simulink model "ADCS_Simulator"  (R2025b)
settings: Solver=ode4  StartTime=0.0  StopTime=tspan  FixedStep=baseRate  RelTol=1e-3
values from neighbouring files (symbols this model uses):
  A_list = [10*30; 10*30; 10*10; 10*30; 10*30; 10*10] * 1e-04    [adcsInitializer.m]
  A_w = eye(3)    [adcsInitializer.m]
  CD = 2.3    [adcsInitializer.m]
  COP = [xAxis/2   0          0 ... (first row only)    [adcsInitializer.m]
  dt = 0.5    [adcsInitializer.m]
  dYear = decyear(YYYY,MM,DD)    [adcsInitializer.m]
  eta = 0.3    [adcsInitializer.m]
  J_body = [ I_xx  I_xy  I_xz ... (first row only)    [adcsInitializer.m]
  mag_moment = [0.005; 0.005; 0.005]    [adcsInitializer.m]
  mu = 398600.4418    [adcsInitializer.m]    (also in montecarlo.m = mean(W,2))
  n_list = [1 0 0; 0 1 0; 0 0 1; -1 0 0; 0 -1 0; 0 0 -1]    [adcsInitializer.m]
  p = 0.00000451    (= 4.51e-06)    [adcsInitializer.m]
  R = blkdiag(sigma_S^2*eye(3), sigma_B^2*eye(3))    [adcsInitializer.m]
  rE = 6378.14    [adcsInitializer.m]
  sigma_b = deg2rad(0.04)/3600    [adcsInitializer.m]
  sigma_B = 0.001    [adcsInitializer.m]
  sigma_g = deg2rad(0.1)/sqrt(3600)    [adcsInitializer.m]
  sigma_S = deg2rad(0.01)    [adcsInitializer.m]
  T = 1    [adcsInitializer.m]
  wE = [0 0 15.04*(pi/180)*(1/3600)]    [adcsInitializer.m]
  wW_1 = 0    [adcsInitializer.m]
  wW_2 = 0    [adcsInitializer.m]
  wW_3 = 0    [adcsInitializer.m]
undefined symbols (not defined in the file or in its folder): ar, controlMode, ext_torque, J_wheels, K_d, K_p, K_w, n, period, pointingMode, q1_ini, q2_ini, q3_ini, q4_ini, r_I_ini, sigmaGPS, turns, useFilter, v_I_ini, wB_1, wB_2, wB_3
libraries: simulink_extras x12
(part 1 of 2)
settings Model: Creator=nimis  LastModifiedBy=nimis

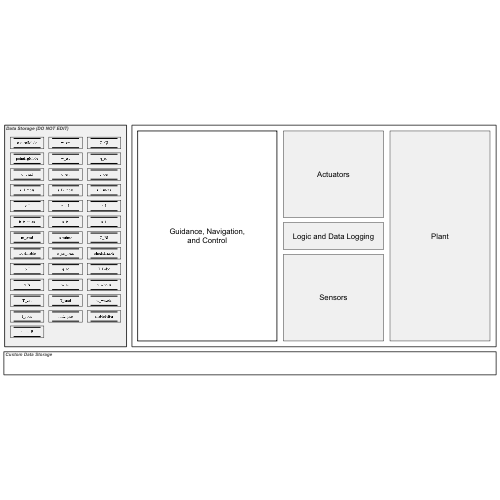
[thumbnail: Simulink's stored preview of the top-level diagram]
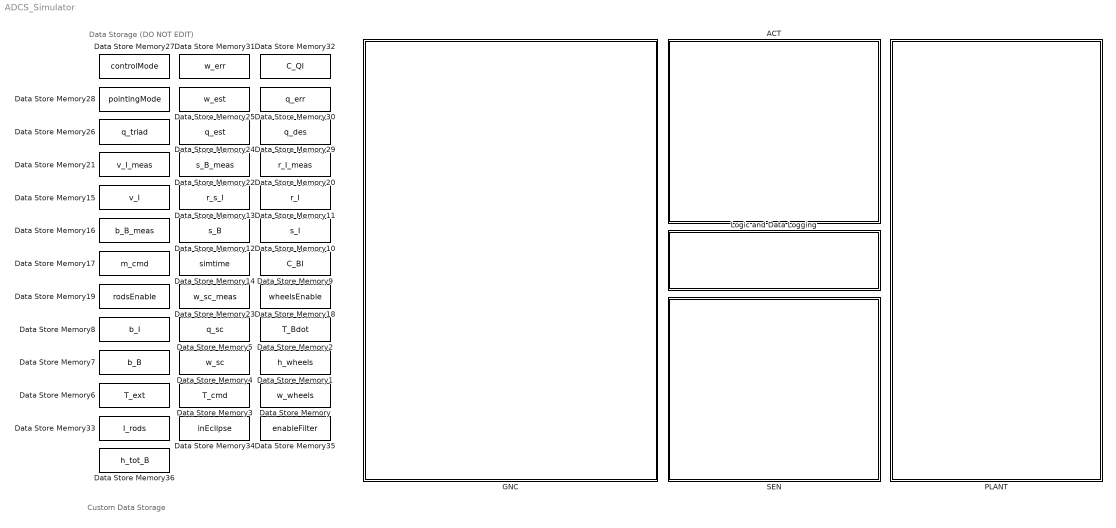
== system ADCS_Simulator ==
  note: Custom Data Storage
  note: Data Storage (DO NOT EDIT)
  ACT : Subsystem
      mask Display: disp('Actuators');
  Data Store Memory : DataStoreMemory  DataStoreName=w_wheels  WriteAfterWriteMsg=warning  InitialValue=[0;0;0]  ShowAdditionalParam=off
  Data Store Memory1 : DataStoreMemory  DataStoreName=h_wheels  WriteAfterWriteMsg=warning  InitialValue=[0;0;0]  ShowAdditionalParam=off
  Data Store Memory10 : DataStoreMemory  DataStoreName=s_I  WriteAfterWriteMsg=warning  InitialValue=[0;0;0]  ShowAdditionalParam=off
  Data Store Memory11 : DataStoreMemory  DataStoreName=r_I  WriteAfterWriteMsg=warning  InitialValue=r_I_ini  ShowAdditionalParam=off
  Data Store Memory12 : DataStoreMemory  DataStoreName=s_B  WriteAfterWriteMsg=warning  InitialValue=[0;0;0]  ShowAdditionalParam=off
  Data Store Memory13 : DataStoreMemory  DataStoreName=r_s_I  WriteAfterWriteMsg=warning  InitialValue=[0;0;0]  ShowAdditionalParam=off
  Data Store Memory14 : DataStoreMemory  DataStoreName=simtime  WriteAfterWriteMsg=warning  ShowAdditionalParam=off
  Data Store Memory15 : DataStoreMemory  DataStoreName=v_I  WriteAfterWriteMsg=warning  InitialValue=v_I_ini  ShowAdditionalParam=off
  Data Store Memory16 : DataStoreMemory  DataStoreName=b_B_meas  WriteAfterWriteMsg=warning  InitialValue=[0;0;0]  ShowAdditionalParam=off
  Data Store Memory17 : DataStoreMemory  DataStoreName=m_cmd  WriteAfterWriteMsg=warning  InitialValue=[0;0;0]  ShowAdditionalParam=off
  Data Store Memory18 : DataStoreMemory  DataStoreName=wheelsEnable  WriteAfterWriteMsg=warning  ShowAdditionalParam=off
  Data Store Memory19 : DataStoreMemory  DataStoreName=rodsEnable  WriteAfterWriteMsg=warning  InitialValue=1  ShowAdditionalParam=off
  Data Store Memory2 : DataStoreMemory  DataStoreName=T_Bdot  WriteAfterWriteMsg=warning  InitialValue=[0;0;0]  ShowAdditionalParam=off
  Data Store Memory20 : DataStoreMemory  DataStoreName=r_I_meas  WriteAfterWriteMsg=warning  InitialValue=r_I_ini  ShowAdditionalParam=off
  Data Store Memory21 : DataStoreMemory  DataStoreName=v_I_meas  WriteAfterWriteMsg=warning  InitialValue=v_I_ini  ShowAdditionalParam=off
  Data Store Memory22 : DataStoreMemory  DataStoreName=s_B_meas  WriteAfterWriteMsg=warning  InitialValue=[0;0;0]  ShowAdditionalParam=off
  Data Store Memory23 : DataStoreMemory  DataStoreName=w_sc_meas  WriteAfterWriteMsg=warning  InitialValue=[wB_1; wB_2; wB_3]*(pi/180)  ShowAdditionalParam=off
  Data Store Memory24 : DataStoreMemory  DataStoreName=q_est  WriteAfterWriteMsg=warning  InitialValue=[q1_ini; q2_ini; q3_ini; q4_ini]  ShowAdditionalParam=off
  Data Store Memory25 : DataStoreMemory  DataStoreName=w_est  WriteAfterWriteMsg=warning  InitialValue=[wB_1; wB_2; wB_3]*(pi/180)  ShowAdditionalParam=off
  Data Store Memory26 : DataStoreMemory  DataStoreName=q_triad  WriteAfterWriteMsg=warning  InitialValue=[q1_ini; q2_ini; q3_ini; q4_ini]  ShowAdditionalParam=off
  Data Store Memory27 : DataStoreMemory  DataStoreName=controlMode  WriteAfterWriteMsg=warning  InitialValue=controlMode  ShowAdditionalParam=off
  Data Store Memory28 : DataStoreMemory  DataStoreName=pointingMode  WriteAfterWriteMsg=warning  InitialValue=pointingMode  ShowAdditionalParam=off
  Data Store Memory29 : DataStoreMemory  DataStoreName=q_des  WriteAfterWriteMsg=warning  InitialValue=[0;0;0;0]  ShowAdditionalParam=off
  Data Store Memory3 : DataStoreMemory  DataStoreName=T_cmd  WriteAfterWriteMsg=warning  InitialValue=[0;0;0]  ShowAdditionalParam=off
  Data Store Memory30 : DataStoreMemory  DataStoreName=q_err  WriteAfterWriteMsg=warning  InitialValue=[0;0;0;1]  ShowAdditionalParam=off
  Data Store Memory31 : DataStoreMemory  DataStoreName=w_err  WriteAfterWriteMsg=warning  InitialValue=[0;0;0]  ShowAdditionalParam=off
  Data Store Memory32 : DataStoreMemory  DataStoreName=C_QI  WriteAfterWriteMsg=warning  InitialValue=eye(3)  ShowAdditionalParam=off
  Data Store Memory33 : DataStoreMemory  DataStoreName=I_rods  WriteAfterWriteMsg=warning  InitialValue=[0;0;0]  ShowAdditionalParam=off
  Data Store Memory34 : DataStoreMemory  DataStoreName=inEclipse  WriteAfterWriteMsg=warning  ShowAdditionalParam=off
  Data Store Memory35 : DataStoreMemory  DataStoreName=enableFilter  WriteAfterWriteMsg=warning  InitialValue=double(useFilter)  ShowAdditionalParam=off
      settings: LockScale=on
  Data Store Memory36 : DataStoreMemory  DataStoreName=h_tot_B  WriteAfterWriteMsg=warning  InitialValue=[0;0;0]  ShowAdditionalParam=off
  Data Store Memory4 : DataStoreMemory  DataStoreName=w_sc  WriteAfterWriteMsg=warning  InitialValue=[wB_1; wB_2; wB_3]*(pi/180)  ShowAdditionalParam=off
  Data Store Memory5 : DataStoreMemory  DataStoreName=q_sc  WriteAfterWriteMsg=warning  InitialValue=[q1_ini; q2_ini; q3_ini; q4_ini]  ShowAdditionalParam=off
  Data Store Memory6 : DataStoreMemory  DataStoreName=T_ext  WriteAfterWriteMsg=warning  InitialValue=[0;0;0]  ShowAdditionalParam=off
  Data Store Memory7 : DataStoreMemory  DataStoreName=b_B  WriteAfterWriteMsg=warning  InitialValue=[0;0;0]  ShowAdditionalParam=off
  Data Store Memory8 : DataStoreMemory  DataStoreName=b_I  WriteAfterWriteMsg=warning  InitialValue=[0;0;0]  ShowAdditionalParam=off
  Data Store Memory9 : DataStoreMemory  DataStoreName=C_BI  WriteAfterWriteMsg=warning  InitialValue=eye(3)  ShowAdditionalParam=off
  GNC : Subsystem  TreatAsAtomicUnit=on  SystemSampleTime=dt
      mask Display: disp('Guidance, Navigation,\nand Control');
  Logic and Data Logging : Subsystem
      mask Display: disp('Logic and Data Logging');
  PLANT : Subsystem
      mask Display: disp('Plant');
  SEN : Subsystem
      mask Display: disp('Sensors');

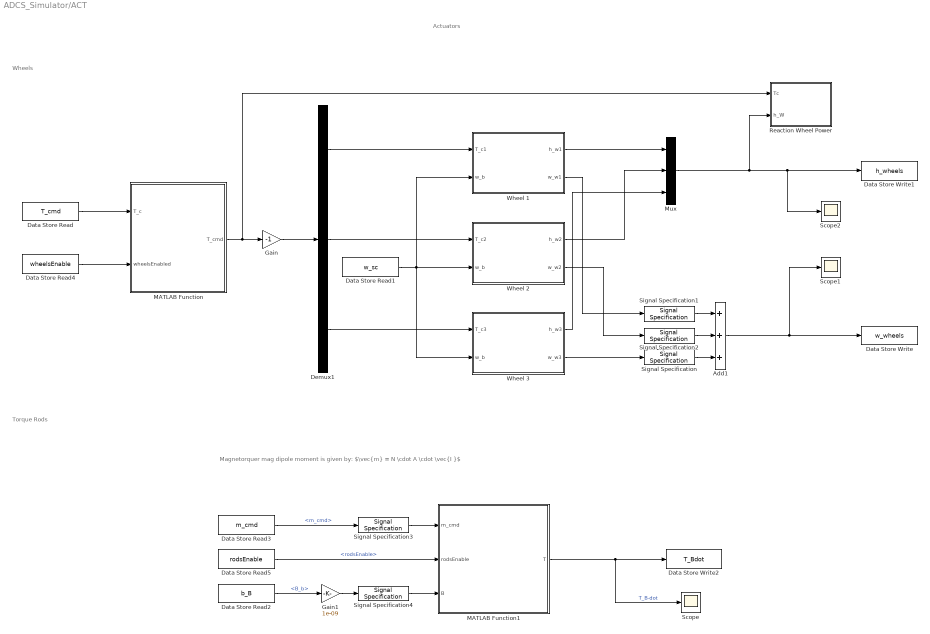
== system ADCS_Simulator/ACT ==
  note: Torque Rods
  note: Wheels
  note: Actuators
  note: Magnetorquer mag dipole moment is given by:
      | $\vec{m} = N \cdot A \cdot \vec{I }$
  Add1 : Sum  Inputs=+++
  Data Store Read : DataStoreRead  DataStoreName=T_cmd  IndexOptions=Index vector (dialog)  Indices=1  OutputSizes=1
  Data Store Read1 : DataStoreRead  DataStoreName=w_sc  IndexOptions=Index vector (dialog)  Indices=1  OutputSizes=1
  Data Store Read2 : DataStoreRead  DataStoreName=b_B  IndexOptions=Index vector (dialog)  Indices=1  OutputSizes=1
  Data Store Read3 : DataStoreRead  DataStoreName=m_cmd  IndexOptions=Index vector (dialog)  Indices=1  OutputSizes=1
  Data Store Read4 : DataStoreRead  DataStoreName=wheelsEnable  IndexOptions=Index vector (dialog)  Indices=1  OutputSizes=1
  Data Store Read5 : DataStoreRead  DataStoreName=rodsEnable  IndexOptions=Index vector (dialog)  Indices=1  OutputSizes=1
  Data Store Write : DataStoreWrite  DataStoreName=w_wheels  IndexOptions=Index vector (dialog)  Indices=1  OutputSizes=1
  Data Store Write1 : DataStoreWrite  DataStoreName=h_wheels  IndexOptions=Index vector (dialog)  Indices=1  OutputSizes=1
  Data Store Write2 : DataStoreWrite  DataStoreName=T_Bdot  IndexOptions=Index vector (dialog)  Indices=1  OutputSizes=1
  Demux1 : Demux  Outputs=3
  Gain : Gain  Gain=-1
  Gain1 : Gain  Gain=1e-09
  MATLAB Function : MATLAB Function  TreatAsAtomicUnit=on
  MATLAB Function1 : MATLAB Function  TreatAsAtomicUnit=on
  Mux : Mux  Inputs=3
  Reaction Wheel Power : Subsystem
  Scope : Scope
      settings: ActiveDisplayYMinimum=-1  ActiveDisplayYMaximum=1  DataLoggingVariableName=ScopeData2
  Scope1 : Scope
      settings: ActiveDisplayYMinimum=-0.2676  ActiveDisplayYMaximum=2.40696
  Scope2 : Scope
      settings: ActiveDisplayYMinimum=-0.00052  ActiveDisplayYMaximum=0.00026
  Signal Specification{,1..4} (5 alike) : SignalSpecification  Dimensions=[3,1]
  Wheel 1 : Subsystem
  Wheel 2 : Subsystem
  Wheel 3 : Subsystem
  wires:
  Data Store Read1/1 -> Wheel 1/2(w_b), Wheel 2/2(w_b), Wheel 3/2(w_b)
  Gain/1 -> Demux1/1
  Wheel 1/2(w_w1) -> Signal Specification1/1
  Demux1/2 -> Wheel 2/1(T_c2)
  Data Store Read4/1 -> MATLAB Function/2(wheelsEnabled)
  Wheel 3/1(h_w3) -> Mux/3
  Wheel 1/1(h_w1) -> Mux/1
  Demux1/1 -> Wheel 1/1(T_c1)
  Data Store Read/1 -> MATLAB Function/1(T_c)
  Signal Specification1/1 -> Add1/1
  Signal Specification2/1 -> Add1/2
  Add1/1 -> Data Store Write/1, Scope1/1
  Wheel 2/1(h_w2) -> Mux/2
  Mux/1 -> Scope2/1, Data Store Write1/1, Reaction Wheel Power/2(h_W)
  Wheel 3/2(w_w3) -> Signal Specification/1
  Demux1/3 -> Wheel 3/1(T_c3)
  Wheel 2/2(w_w2) -> Signal Specification2/1
  MATLAB Function/1(T_cmd) -> Gain/1, Reaction Wheel Power/1(Tc)
  Signal Specification/1 -> Add1/3
  Data Store Read3/1 -> Signal Specification3/1  "<m_cmd>"
  Data Store Read2/1 -> Gain1/1  "<B_b>"
  Signal Specification4/1 -> MATLAB Function1/3(B)
  Signal Specification3/1 -> MATLAB Function1/1(m_cmd)
  Data Store Read5/1 -> MATLAB Function1/2(rodsEnable)  "<rodsEnable>"
  MATLAB Function1/1(T) -> Data Store Write2/1, Scope/1  "T_B-dot"
  Gain1/1 -> Signal Specification4/1

== system ADCS_Simulator/GNC ==
  note: Guidance, Navigation, and Control
  Control : Subsystem
  Data Store Write10 : DataStoreWrite  DataStoreName=m_cmd  IndexOptions=Index vector (dialog)  Indices=1  OutputSizes=1
  Data Store Write9 : DataStoreWrite  DataStoreName=T_cmd  IndexOptions=Index vector (dialog)  Indices=1  OutputSizes=1
  Guidance : Subsystem
  Navigation : Subsystem
  wires:
  Navigation/1(q_est) -> Guidance/1(q_body)
  Navigation/2(w_est) -> Guidance/2(w_body)
  Control/1(T_cmd) -> Data Store Write9/1
  Control/2(m_cmd) -> Data Store Write10/1

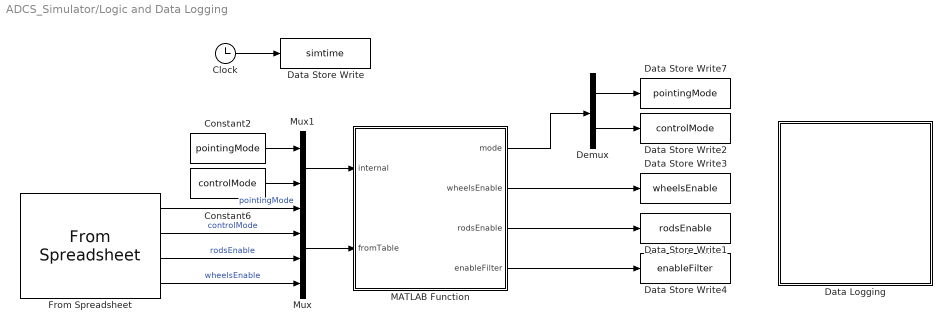
== system ADCS_Simulator/Logic and Data Logging ==
  Clock : Clock
  Constant2 : Constant  Value=pointingMode
  Constant6 : Constant  Value=controlMode
  Data Logging : Subsystem
  Data Store Write : DataStoreWrite  DataStoreName=simtime  IndexOptions=Index vector (dialog)  Indices=1  OutputSizes=1
  Data Store Write1 : DataStoreWrite  DataStoreName=rodsEnable  IndexOptions=Index vector (dialog)  Indices=1  OutputSizes=1
  Data Store Write2 : DataStoreWrite  DataStoreName=controlMode  IndexOptions=Index vector (dialog)  Indices=1  OutputSizes=1
  Data Store Write3 : DataStoreWrite  DataStoreName=wheelsEnable  IndexOptions=Index vector (dialog)  Indices=1  OutputSizes=1
  Data Store Write4 : DataStoreWrite  DataStoreName=enableFilter  IndexOptions=Index vector (dialog)  Indices=1  OutputSizes=1
  Data Store Write7 : DataStoreWrite  DataStoreName=pointingMode  IndexOptions=Index vector (dialog)  Indices=1  OutputSizes=1
  Demux : Demux  Outputs=2
  From Spreadsheet : FromSpreadsheet  FileName=controlCommand.xlsx  SheetName=commands  Range=B1:F1000  InterpolationWithinTimeRange=Zero order hold  ExtrapolationAfterLastDataPoint=Hold last value
  MATLAB Function : MATLAB Function  TreatAsAtomicUnit=on
  Mux : Mux
  Mux1 : Mux  Inputs=2
  wires:
  Clock/1 -> Data Store Write/1
  MATLAB Function/3(rodsEnable) -> Data Store Write1/1
  Mux/1 -> MATLAB Function/2(fromTable)
  From Spreadsheet/1 -> Mux/1  "pointingMode"
  Mux1/1 -> MATLAB Function/1(internal)
  MATLAB Function/2(wheelsEnable) -> Data Store Write3/1
  From Spreadsheet/3 -> Mux/3  "rodsEnable"
  From Spreadsheet/2 -> Mux/2  "controlMode"
  Constant2/1 -> Mux1/1
  Constant6/1 -> Mux1/2
  Demux/1 -> Data Store Write7/1
  Demux/2 -> Data Store Write2/1
  MATLAB Function/4(enableFilter) -> Data Store Write4/1
  From Spreadsheet/4 -> Mux/4  "wheelsEnable"
  MATLAB Function/1(mode) -> Demux/1

== system ADCS_Simulator/PLANT ==
  note: PLANT
  Data Store Read3 : DataStoreRead  DataStoreName=h_wheels  IndexOptions=Index vector (dialog)  Indices=1  OutputSizes=1
  Data Store Read4 : DataStoreRead  DataStoreName=T_Bdot  IndexOptions=Index vector (dialog)  Indices=1  OutputSizes=1
  Data Store Read5 : DataStoreRead  DataStoreName=T_ext  IndexOptions=Index vector (dialog)  Indices=1  OutputSizes=1
  Data Store Write : DataStoreWrite  DataStoreName=T_ext  IndexOptions=Index vector (dialog)  Indices=1  OutputSizes=1
  Data Store Write3 : DataStoreWrite  DataStoreName=w_sc  IndexOptions=Index vector (dialog)  Indices=1  OutputSizes=1
  Data Store Write4 : DataStoreWrite  DataStoreName=q_sc  IndexOptions=Index vector (dialog)  Indices=1  OutputSizes=1
  ENV : Subsystem  Priority=4  VariantControl=ext_torque == true
  Orbit Propator : Subsystem  Priority=3
  Spacecraft Dynamics : Subsystem  Priority=1
  Spacecraft Kinematics : Subsystem  Priority=2
  wires:
  ENV/1(T_ext) -> Data Store Write/1
  Data Store Read5/1 -> Spacecraft Dynamics/2(T_ext)
  Spacecraft Kinematics/1(q) -> Data Store Write4/1
  Data Store Read3/1 -> Spacecraft Dynamics/1(h_w)
  Spacecraft Dynamics/1(w_b) -> Data Store Write3/1, Spacecraft Kinematics/1(w)
  Data Store Read4/1 -> Spacecraft Dynamics/3(T_Bdot)

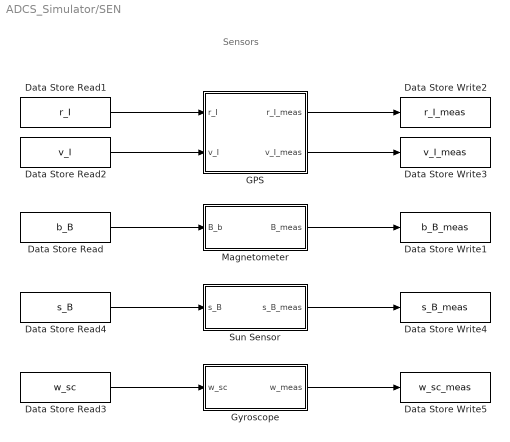
== system ADCS_Simulator/SEN ==
  note: Sensors
  Data Store Read : DataStoreRead  DataStoreName=b_B  IndexOptions=Index vector (dialog)  Indices=1  OutputSizes=1
  Data Store Read1 : DataStoreRead  DataStoreName=r_I  IndexOptions=Index vector (dialog)  Indices=1  OutputSizes=1
  Data Store Read2 : DataStoreRead  DataStoreName=v_I  IndexOptions=Index vector (dialog)  Indices=1  OutputSizes=1
  Data Store Read3 : DataStoreRead  DataStoreName=w_sc  IndexOptions=Index vector (dialog)  Indices=1  OutputSizes=1
  Data Store Read4 : DataStoreRead  DataStoreName=s_B  IndexOptions=Index vector (dialog)  Indices=1  OutputSizes=1
  Data Store Write1 : DataStoreWrite  DataStoreName=b_B_meas  IndexOptions=Index vector (dialog)  Indices=1  OutputSizes=1
  Data Store Write2 : DataStoreWrite  DataStoreName=r_I_meas  IndexOptions=Index vector (dialog)  Indices=1  OutputSizes=1
  Data Store Write3 : DataStoreWrite  DataStoreName=v_I_meas  IndexOptions=Index vector (dialog)  Indices=1  OutputSizes=1
  Data Store Write4 : DataStoreWrite  DataStoreName=s_B_meas  IndexOptions=Index vector (dialog)  Indices=1  OutputSizes=1
  Data Store Write5 : DataStoreWrite  DataStoreName=w_sc_meas  IndexOptions=Index vector (dialog)  Indices=1  OutputSizes=1
  GPS : Subsystem
  Gyroscope : Subsystem
  Magnetometer : Subsystem
  Sun Sensor : Subsystem
  wires:
  GPS/1(r_I_meas) -> Data Store Write2/1
  GPS/2(v_I_meas) -> Data Store Write3/1
  Magnetometer/1(B_meas) -> Data Store Write1/1
  Sun Sensor/1(s_B_meas) -> Data Store Write4/1
  Gyroscope/1(w_meas) -> Data Store Write5/1
  Data Store Read1/1 -> GPS/1(r_I)
  Data Store Read2/1 -> GPS/2(v_I)
  Data Store Read/1 -> Magnetometer/1(B_b)
  Data Store Read4/1 -> Sun Sensor/1(s_B)
  Data Store Read3/1 -> Gyroscope/1(w_sc)

== system ADCS_Simulator/ACT/Reaction Wheel Power ==
  Tc : Inport
  h_W : Inport  Port=2
  MATLAB Function3 : MATLAB Function  TreatAsAtomicUnit=on
  Scope2 : Scope
      settings: ActiveDisplayYMinimum=-170.39311  ActiveDisplayYMaximum=1533.53798  DataLoggingVariableName=ScopeData2
  Scope4 : Scope
      settings: ActiveDisplayYMinimum=-0.0048  ActiveDisplayYMaximum=0.04316
  To Workspace : ToWorkspace  VariableName=Prw  SampleTime=-1
  Unit Delay : UnitDelay  InitialCondition=zeros(3,1)  SampleTime=-1  HasFrameUpgradeWarning=on
  wires:
  MATLAB Function3/1(Prw) -> To Workspace/1, Scope4/1
  Tc/1 -> MATLAB Function3/1(Tc)
  MATLAB Function3/2(Ptotal) -> Unit Delay/1, Scope2/1
  h_W/1 -> MATLAB Function3/2(h_W)
  Unit Delay/1 -> MATLAB Function3/3(P_pre)

== system ADCS_Simulator/ACT/Wheel 1 ==
  T_c1 : Inport
  w_b : Inport  Port=2
  Constant1 : Constant  Value=A_w
  Constant2 : Constant  Value=J_wheels
  Integrator1 : Integrator  InitialCondition=wW_1*J_wheels
  MATLAB Function1 : MATLAB Function  TreatAsAtomicUnit=on
  Reshape : Reshape  OutputDimensionality=Column vector (2-D)
  Transfer Fcn : TransferFcn  Commented=on  Numerator=[2.11e04]  Denominator=[J_wheels 1 0]
  Transfer Fcn (with initial states) : simulink_extras/Additional Linear/Transfer Fcn (with initial states)  Commented=on  N=[1]  D="[T  1]"  X0=wW_1*J_wheels
  h_w1 : Outport
  w_w1 : Outport  Port=2
  wires:
  Constant2/1 -> MATLAB Function1/1(J_w)
  T_c1/1 -> Integrator1/1
  w_b/1 -> Reshape/1
  Constant1/1 -> MATLAB Function1/4(A_w)
  MATLAB Function1/1(h_wi) -> h_w1/1
  MATLAB Function1/2(w_wi) -> w_w1/1
  Integrator1/1 -> MATLAB Function1/2(h_w)
  Reshape/1 -> MATLAB Function1/3(wB)

== system ADCS_Simulator/ACT/Wheel 2 ==
  T_c2 : Inport
  w_b : Inport  Port=2
  Constant2 : Constant  Value=A_w
  Constant3 : Constant  Value=J_wheels
  Integrator1 : Integrator  InitialCondition=wW_2*J_wheels
  MATLAB Function1 : MATLAB Function  TreatAsAtomicUnit=on
  Reshape : Reshape  OutputDimensionality=Column vector (2-D)
  Transfer Fcn : TransferFcn  Commented=on  Numerator=[2.11e04]  Denominator=[J_wheels 1 0]
  Transfer Fcn (with initial states) : simulink_extras/Additional Linear/Transfer Fcn (with initial states)  Commented=on  N=[1]  D="[T  1]"  X0=wW_2*J_wheels
  h_w2 : Outport
  w_w2 : Outport  Port=2
  wires:
  Constant2/1 -> MATLAB Function1/4(A_w)
  T_c2/1 -> Integrator1/1
  Constant3/1 -> MATLAB Function1/1(J_w)
  MATLAB Function1/2(w_wi) -> w_w2/1
  Integrator1/1 -> MATLAB Function1/2(h_w)
  MATLAB Function1/1(h_wi) -> h_w2/1
  w_b/1 -> Reshape/1
  Reshape/1 -> MATLAB Function1/3(wB)

== system ADCS_Simulator/ACT/Wheel 3 ==
  T_c3 : Inport
  w_b : Inport  Port=2
  Constant2 : Constant  Value=A_w
  Constant3 : Constant  Value=J_wheels
  Integrator1 : Integrator  InitialCondition=wW_3*J_wheels
  MATLAB Function1 : MATLAB Function  TreatAsAtomicUnit=on
  Reshape : Reshape  OutputDimensionality=Column vector (2-D)
  Transfer Fcn : TransferFcn  Commented=on  Numerator=[2.11e04]  Denominator=[J_wheels 1 0]
  Transfer Fcn (with initial states) : simulink_extras/Additional Linear/Transfer Fcn (with initial states)  Commented=on  N=[1]  D="[T  1]"  X0=wW_3*J_wheels
  h_w3 : Outport
  w_w3 : Outport  Port=2
  wires:
  Constant2/1 -> MATLAB Function1/4(A_w)
  T_c3/1 -> Integrator1/1
  Constant3/1 -> MATLAB Function1/1(J_w)
  MATLAB Function1/2(w_wi) -> w_w3/1
  Integrator1/1 -> MATLAB Function1/2(h_w)
  MATLAB Function1/1(h_wi) -> h_w3/1
  w_b/1 -> Reshape/1
  Reshape/1 -> MATLAB Function1/3(wB)

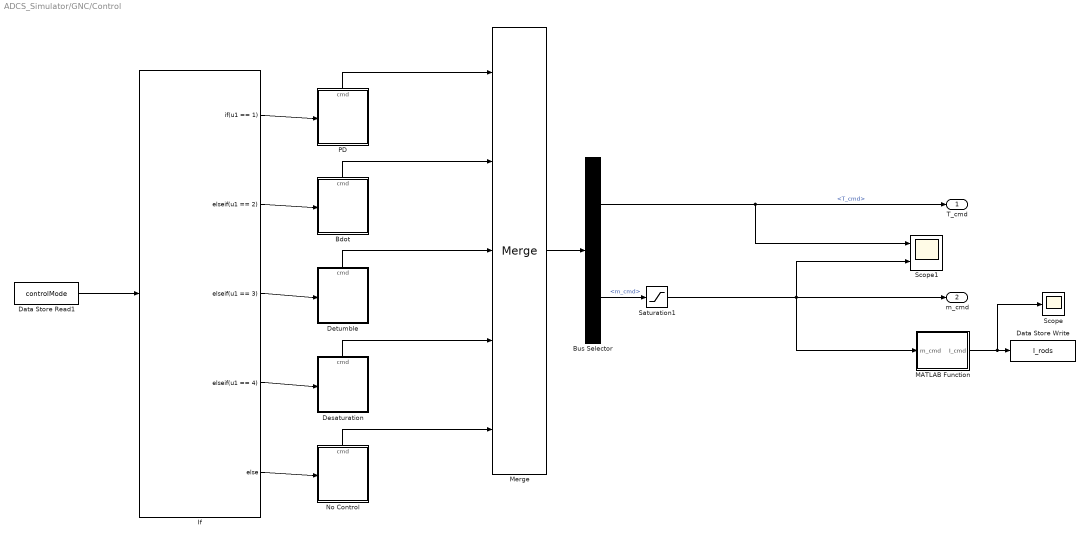
== system ADCS_Simulator/GNC/Control ==
  Bdot : Subsystem  TreatAsAtomicUnit=on
  Bus Selector : BusSelector  OutputSignals=T_cmd,m_cmd
  Data Store Read1 : DataStoreRead  DataStoreName=controlMode  IndexOptions=Index vector (dialog)  Indices=1  OutputSizes=1
  Data Store Write : DataStoreWrite  DataStoreName=I_rods  IndexOptions=Index vector (dialog)  Indices=1  OutputSizes=1
  Desaturation : Subsystem  TreatAsAtomicUnit=on
  Detumble : Subsystem  TreatAsAtomicUnit=on
  If : If  IfExpression=u1 == 1  ElseIfExpressions=u1 == 2, u1 == 3, u1 == 4
  MATLAB Function : MATLAB Function  TreatAsAtomicUnit=on
  Merge : Merge  Inputs=5
  No Control : Subsystem  TreatAsAtomicUnit=on
  "PD " : Subsystem  TreatAsAtomicUnit=on
  Saturation1 : Saturate  UpperLimit=0.2  LowerLimit=-0.2
  Scope : Scope
      settings: ActiveDisplayYMinimum=-1  ActiveDisplayYMaximum=1  DataLoggingVariableName=ScopeData2
  Scope1 : Scope  NumInputPorts=2
      settings: ActiveDisplayYMinimum=-7.0811470476357021E-5  ActiveDisplayYMaximum=7.7475119642045185E-5  DataLoggingVariableName=ScopeData4
  T_cmd : Outport
  m_cmd : Outport  Port=2
  wires:
  If/1 -> "PD "/Action
  If/2 -> Bdot/Action
  If/3 -> Detumble/Action
  If/4 -> Desaturation/Action
  If/5 -> No Control/Action
  Data Store Read1/1 -> If/1
  "PD "/1(cmd) -> Merge/1
  Bdot/1(cmd) -> Merge/2
  Detumble/1(cmd) -> Merge/3
  Desaturation/1(cmd) -> Merge/4
  No Control/1(cmd) -> Merge/5
  Merge/1 -> Bus Selector/1
  Saturation1/1 -> MATLAB Function/1(m_cmd), Scope1/2, m_cmd/1
  Bus Selector/2 -> Saturation1/1  "<m_cmd>"
  Bus Selector/1 -> T_cmd/1, Scope1/1  "<T_cmd>"
  MATLAB Function/1(I_cmd) -> Scope/1, Data Store Write/1

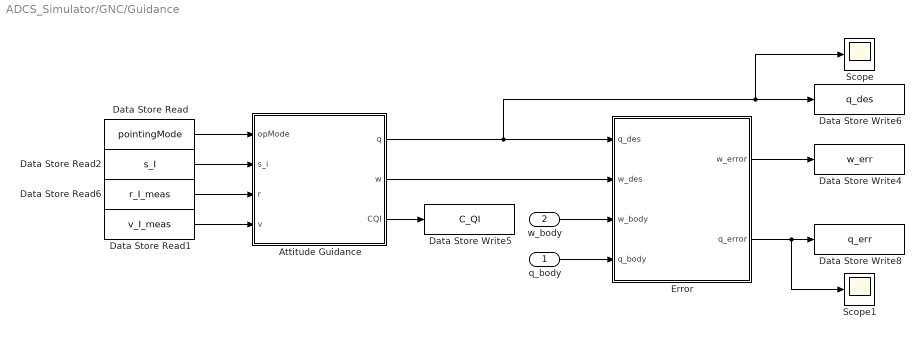
== system ADCS_Simulator/GNC/Guidance ==
  q_body : Inport
  w_body : Inport  Port=2
  Attitude Guidance : MATLAB Function  TreatAsAtomicUnit=on
  Data Store Read : DataStoreRead  DataStoreName=pointingMode  IndexOptions=Index vector (dialog)  Indices=1  OutputSizes=1
  Data Store Read1 : DataStoreRead  DataStoreName=v_I_meas  IndexOptions=Index vector (dialog)  Indices=1  OutputSizes=1
  Data Store Read2 : DataStoreRead  DataStoreName=s_I  IndexOptions=Index vector (dialog)  Indices=1  OutputSizes=1
  Data Store Read6 : DataStoreRead  DataStoreName=r_I_meas  IndexOptions=Index vector (dialog)  Indices=1  OutputSizes=1
  Data Store Write4 : DataStoreWrite  DataStoreName=w_err  IndexOptions=Index vector (dialog)  Indices=1  OutputSizes=1
  Data Store Write5 : DataStoreWrite  DataStoreName=C_QI  IndexOptions=Index vector (dialog)  Indices=1  OutputSizes=1
  Data Store Write6 : DataStoreWrite  DataStoreName=q_des  IndexOptions=Index vector (dialog)  Indices=1  OutputSizes=1
  Data Store Write8 : DataStoreWrite  DataStoreName=q_err  IndexOptions=Index vector (dialog)  Indices=1  OutputSizes=1
  Error : Subsystem
  Scope : Scope
      settings: ActiveDisplayYMinimum=-1.056652169354914  ActiveDisplayYMaximum=0.82334453801197993
  Scope1 : Scope
      settings: ActiveDisplayYMinimum=-1  ActiveDisplayYMaximum=1  DataLoggingVariableName=ScopeData2
  wires:
  Error/2(q_error) -> Scope1/1, Data Store Write8/1
  Data Store Read/1 -> Attitude Guidance/1(opMode)
  Data Store Read6/1 -> Attitude Guidance/3(r)
  Data Store Read2/1 -> Attitude Guidance/2(s_i)
  Error/1(w_error) -> Data Store Write4/1
  Attitude Guidance/3(CQI) -> Data Store Write5/1
  q_body/1 -> Error/4(q_body)
  Data Store Read1/1 -> Attitude Guidance/4(v)
  w_body/1 -> Error/3(w_body)
  Attitude Guidance/2(w) -> Error/2(w_des)
  Attitude Guidance/1(q) -> Error/1(q_des), Scope/1, Data Store Write6/1

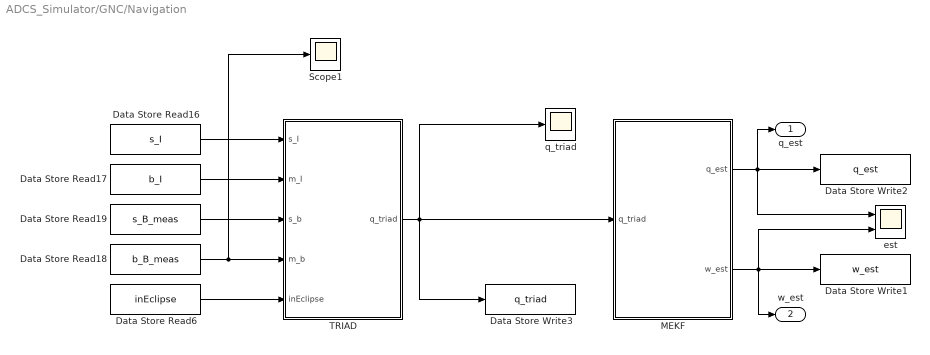
== system ADCS_Simulator/GNC/Navigation ==
  Data Store Read16 : DataStoreRead  DataStoreName=s_I  IndexOptions=Index vector (dialog)  Indices=1  OutputSizes=1
  Data Store Read17 : DataStoreRead  DataStoreName=b_I  IndexOptions=Index vector (dialog)  Indices=1  OutputSizes=1
  Data Store Read18 : DataStoreRead  DataStoreName=b_B_meas  IndexOptions=Index vector (dialog)  Indices=1  OutputSizes=1
  Data Store Read19 : DataStoreRead  DataStoreName=s_B_meas  IndexOptions=Index vector (dialog)  Indices=1  OutputSizes=1
  Data Store Read6 : DataStoreRead  DataStoreName=inEclipse  IndexOptions=Index vector (dialog)  Indices=1  OutputSizes=1
  Data Store Write1 : DataStoreWrite  DataStoreName=w_est  IndexOptions=Index vector (dialog)  Indices=1  OutputSizes=1
  Data Store Write2 : DataStoreWrite  DataStoreName=q_est  IndexOptions=Index vector (dialog)  Indices=1  OutputSizes=1
  Data Store Write3 : DataStoreWrite  DataStoreName=q_triad  IndexOptions=Index vector (dialog)  Indices=1  OutputSizes=1
  MEKF : Subsystem
  Scope1 : Scope
      settings: ActiveDisplayYMinimum=-14383.00265  ActiveDisplayYMaximum=50097.51975
  TRIAD : MATLAB Function  TreatAsAtomicUnit=on
  est : Scope  NumInputPorts=2
      settings: ActiveDisplayYMinimum=-1.1965212617720182  ActiveDisplayYMaximum=1.242899979906531
  q_triad : Scope
      settings: ActiveDisplayYMinimum=-1.09993445466622  ActiveDisplayYMaximum=1.2333260505184689  DataLoggingVariableName=ScopeData3
  q_est : Outport
  w_est : Outport  Port=2
  wires:
  Data Store Read19/1 -> TRIAD/3(s_b)
  MEKF/2(w_est) -> w_est/1, Data Store Write1/1, est/2
  MEKF/1(q_est) -> q_est/1, Data Store Write2/1, est/1
  Data Store Read18/1 -> Scope1/1, TRIAD/4(m_b)
  Data Store Read17/1 -> TRIAD/2(m_I)
  TRIAD/1(q_triad) -> Data Store Write3/1, q_triad/1, MEKF/1(q_triad)
  Data Store Read16/1 -> TRIAD/1(s_I)
  Data Store Read6/1 -> TRIAD/5(inEclipse)

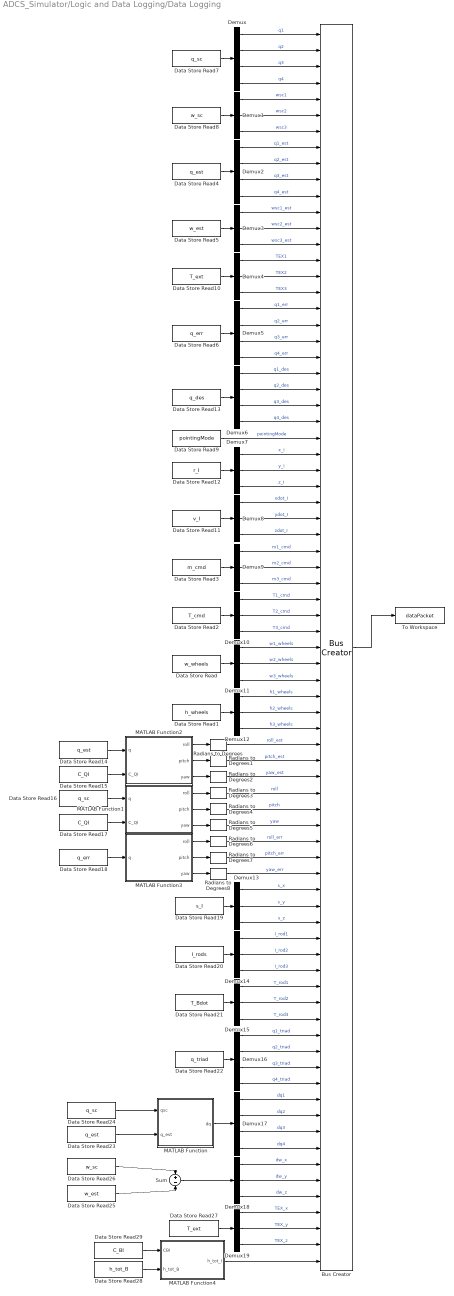
== system ADCS_Simulator/Logic and Data Logging/Data Logging ==
  Bus Creator : BusCreator  Inputs=77
  Data Store Read : DataStoreRead  DataStoreName=w_wheels  IndexOptions=Index vector (dialog)  Indices=1  OutputSizes=1
  Data Store Read1 : DataStoreRead  DataStoreName=h_wheels  IndexOptions=Index vector (dialog)  Indices=1  OutputSizes=1
  Data Store Read10 : DataStoreRead  DataStoreName=T_ext  IndexOptions=Index vector (dialog)  Indices=1  OutputSizes=1
  Data Store Read11 : DataStoreRead  DataStoreName=v_I  IndexOptions=Index vector (dialog)  Indices=1  OutputSizes=1
  Data Store Read12 : DataStoreRead  DataStoreName=r_I  IndexOptions=Index vector (dialog)  Indices=1  OutputSizes=1
  Data Store Read13 : DataStoreRead  DataStoreName=q_des  IndexOptions=Index vector (dialog)  Indices=1  OutputSizes=1
  Data Store Read14 : DataStoreRead  DataStoreName=q_est  IndexOptions=Index vector (dialog)  Indices=1  OutputSizes=1
  Data Store Read15 : DataStoreRead  DataStoreName=C_QI  IndexOptions=Index vector (dialog)  Indices=1  OutputSizes=1
  Data Store Read16 : DataStoreRead  DataStoreName=q_sc  IndexOptions=Index vector (dialog)  Indices=1  OutputSizes=1
  Data Store Read17 : DataStoreRead  DataStoreName=C_QI  IndexOptions=Index vector (dialog)  Indices=1  OutputSizes=1
  Data Store Read18 : DataStoreRead  DataStoreName=q_err  IndexOptions=Index vector (dialog)  Indices=1  OutputSizes=1
  Data Store Read19 : DataStoreRead  DataStoreName=s_I  IndexOptions=Index vector (dialog)  Indices=1  OutputSizes=1
  Data Store Read2 : DataStoreRead  DataStoreName=T_cmd  IndexOptions=Index vector (dialog)  Indices=1  OutputSizes=1
  Data Store Read20 : DataStoreRead  DataStoreName=I_rods  IndexOptions=Index vector (dialog)  Indices=1  OutputSizes=1
  Data Store Read21 : DataStoreRead  DataStoreName=T_Bdot  IndexOptions=Index vector (dialog)  Indices=1  OutputSizes=1
  Data Store Read22 : DataStoreRead  DataStoreName=q_triad  IndexOptions=Index vector (dialog)  Indices=1  OutputSizes=1
  Data Store Read23 : DataStoreRead  DataStoreName=q_est  IndexOptions=Index vector (dialog)  Indices=1  OutputSizes=1
  Data Store Read24 : DataStoreRead  DataStoreName=q_sc  IndexOptions=Index vector (dialog)  Indices=1  OutputSizes=1
  Data Store Read25 : DataStoreRead  DataStoreName=w_est  IndexOptions=Index vector (dialog)  Indices=1  OutputSizes=1
  Data Store Read26 : DataStoreRead  DataStoreName=w_sc  IndexOptions=Index vector (dialog)  Indices=1  OutputSizes=1
  Data Store Read27 : DataStoreRead  DataStoreName=T_ext  IndexOptions=Index vector (dialog)  Indices=1  OutputSizes=1
  Data Store Read28 : DataStoreRead  DataStoreName=h_tot_B  IndexOptions=Index vector (dialog)  Indices=1  OutputSizes=1
  Data Store Read29 : DataStoreRead  DataStoreName=C_BI  IndexOptions=Index vector (dialog)  Indices=1  OutputSizes=1
  Data Store Read3 : DataStoreRead  DataStoreName=m_cmd  IndexOptions=Index vector (dialog)  Indices=1  OutputSizes=1
  Data Store Read4 : DataStoreRead  DataStoreName=q_est  IndexOptions=Index vector (dialog)  Indices=1  OutputSizes=1
  Data Store Read5 : DataStoreRead  DataStoreName=w_est  IndexOptions=Index vector (dialog)  Indices=1  OutputSizes=1
  Data Store Read6 : DataStoreRead  DataStoreName=q_err  IndexOptions=Index vector (dialog)  Indices=1  OutputSizes=1
  Data Store Read7 : DataStoreRead  DataStoreName=q_sc  IndexOptions=Index vector (dialog)  Indices=1  OutputSizes=1
  Data Store Read8 : DataStoreRead  DataStoreName=w_sc  IndexOptions=Index vector (dialog)  Indices=1  OutputSizes=1
  Data Store Read9 : DataStoreRead  DataStoreName=pointingMode  IndexOptions=Index vector (dialog)  Indices=1  OutputSizes=1
  Demux{,2,5..6,16..17} (6 alike) : Demux
  Demux{1,3..4,7..15,18..19} (14 alike) : Demux  Outputs=3
  MATLAB Function : MATLAB Function  TreatAsAtomicUnit=on
  MATLAB Function1 : MATLAB Function  TreatAsAtomicUnit=on
  MATLAB Function2 : MATLAB Function  TreatAsAtomicUnit=on
  MATLAB Function3 : MATLAB Function  TreatAsAtomicUnit=on
  MATLAB Function4 : MATLAB Function  TreatAsAtomicUnit=on
  Radians to Degrees{,1..8} (9 alike) : simulink_extras/Transformations/Radians to Degrees
  Sum : Sum  Inputs=+-
  To Workspace : ToWorkspace  VariableName=dataPacket  SaveFormat=Timeseries  SampleTime=-1
  wires:
  Data Store Read7/1 -> Demux/1
  Demux/1 -> Bus Creator/1  "q1"
  Demux/2 -> Bus Creator/2  "q2"
  Demux/3 -> Bus Creator/3  "q3"
  Demux/4 -> Bus Creator/4  "q4"
  Data Store Read8/1 -> Demux1/1
  Demux1/1 -> Bus Creator/5  "wsc1"
  Demux1/2 -> Bus Creator/6  "wsc2"
  Demux1/3 -> Bus Creator/7  "wsc3"
  Demux2/1 -> Bus Creator/8  "q1_est"
  Demux2/2 -> Bus Creator/9  "q2_est"
  Demux2/3 -> Bus Creator/10  "q3_est"
  Demux2/4 -> Bus Creator/11  "q4_est"
  Data Store Read4/1 -> Demux2/1
  Demux3/1 -> Bus Creator/12  "wsc1_est"
  Demux3/2 -> Bus Creator/13  "wsc2_est"
  Demux3/3 -> Bus Creator/14  "wsc3_est"
  Data Store Read5/1 -> Demux3/1
  Demux4/1 -> Bus Creator/15  "TEX1"
  Demux4/2 -> Bus Creator/16  "TEX2"
  Demux4/3 -> Bus Creator/17  "TEX3"
  Data Store Read10/1 -> Demux4/1
  Demux5/1 -> Bus Creator/18  "q1_err"
  Demux5/2 -> Bus Creator/19  "q2_err"
  Demux5/3 -> Bus Creator/20  "q3_err"
  Demux5/4 -> Bus Creator/21  "q4_err"
  Data Store Read6/1 -> Demux5/1
  Demux6/1 -> Bus Creator/22  "q1_des"
  Demux6/2 -> Bus Creator/23  "q2_des"
  Demux6/3 -> Bus Creator/24  "q3_des"
  Demux6/4 -> Bus Creator/25  "q4_des"
  Data Store Read13/1 -> Demux6/1
  Data Store Read9/1 -> Bus Creator/26  "pointingMode"
  Demux7/1 -> Bus Creator/27  "x_I"
  Demux7/2 -> Bus Creator/28  "y_I"
  Demux7/3 -> Bus Creator/29  "z_I"
  Data Store Read12/1 -> Demux7/1
  Demux8/1 -> Bus Creator/30  "xdot_I"
  Demux8/2 -> Bus Creator/31  "ydot_I"
  Demux8/3 -> Bus Creator/32  "zdot_I"
  Data Store Read11/1 -> Demux8/1
  Demux9/1 -> Bus Creator/33  "m1_cmd"
  Demux9/2 -> Bus Creator/34  "m2_cmd"
  Demux9/3 -> Bus Creator/35  "m3_cmd"
  Data Store Read3/1 -> Demux9/1
  Demux10/1 -> Bus Creator/36  "T1_cmd"
  Demux10/2 -> Bus Creator/37  "T2_cmd"
  Demux10/3 -> Bus Creator/38  "T3_cmd"
  Data Store Read2/1 -> Demux10/1
  Demux11/1 -> Bus Creator/39  "w1_wheels"
  Demux11/2 -> Bus Creator/40  "w2_wheels"
  Demux11/3 -> Bus Creator/41  "w3_wheels"
  Data Store Read/1 -> Demux11/1
  Demux12/1 -> Bus Creator/42  "h1_wheels"
  Demux12/2 -> Bus Creator/43  "h2_wheels"
  Demux12/3 -> Bus Creator/44  "h3_wheels"
  Data Store Read1/1 -> Demux12/1
  Bus Creator/1 -> To Workspace/1
  MATLAB Function2/1(roll) -> Radians to Degrees/1
  MATLAB Function2/3(yaw) -> Radians to Degrees2/1
  MATLAB Function2/2(pitch) -> Radians to Degrees1/1
  Data Store Read14/1 -> MATLAB Function2/1(q)
  Data Store Read15/1 -> MATLAB Function2/2(C_QI)
  Radians to Degrees/1 -> Bus Creator/45  "roll_est"
  Radians to Degrees1/1 -> Bus Creator/46  "pitch_est"
  Radians to Degrees2/1 -> Bus Creator/47  "yaw_est"
  Radians to Degrees5/1 -> Bus Creator/50  "yaw"
  Radians to Degrees4/1 -> Bus Creator/49  "pitch"
  Radians to Degrees3/1 -> Bus Creator/48  "roll"
  Data Store Read17/1 -> MATLAB Function1/2(C_QI)
  Data Store Read16/1 -> MATLAB Function1/1(q)
  MATLAB Function1/2(pitch) -> Radians to Degrees4/1
  MATLAB Function1/3(yaw) -> Radians to Degrees5/1
  MATLAB Function1/1(roll) -> Radians to Degrees3/1
  MATLAB Function3/1(roll) -> Radians to Degrees6/1
  MATLAB Function3/2(pitch) -> Radians to Degrees7/1
  MATLAB Function3/3(yaw) -> Radians to Degrees8/1
  Data Store Read18/1 -> MATLAB Function3/1(q)
  Radians to Degrees6/1 -> Bus Creator/51  "roll_err"
  Radians to Degrees7/1 -> Bus Creator/52  "pitch_err"
  Radians to Degrees8/1 -> Bus Creator/53  "yaw_err"
  Data Store Read19/1 -> Demux13/1
  Demux13/1 -> Bus Creator/54  "s_x"
  Demux13/2 -> Bus Creator/55  "s_y"
  Demux13/3 -> Bus Creator/56  "s_z"
  Data Store Read20/1 -> Demux14/1
  Demux14/1 -> Bus Creator/57  "I_rod1"
  Demux14/2 -> Bus Creator/58  "I_rod2"
  Demux14/3 -> Bus Creator/59  "I_rod3"
  Demux15/1 -> Bus Creator/60  "T_rod1"
  Demux15/2 -> Bus Creator/61  "T_rod2"
  Demux15/3 -> Bus Creator/62  "T_rod3"
  Data Store Read21/1 -> Demux15/1
  Demux16/3 -> Bus Creator/65  "q3_triad"
  Demux16/1 -> Bus Creator/63  "q1_triad"
  Demux16/2 -> Bus Creator/64  "q2_triad"
  Data Store Read22/1 -> Demux16/1
  Demux16/4 -> Bus Creator/66  "q4_triad"
  Demux17/1 -> Bus Creator/67  "dq1"
  Demux17/2 -> Bus Creator/68  "dq2"
  Demux17/3 -> Bus Creator/69  "dq3"
  Demux17/4 -> Bus Creator/70  "dq4"
  Demux18/1 -> Bus Creator/71  "dw_x"
  Demux18/2 -> Bus Creator/72  "dw_y"
  Demux18/3 -> Bus Creator/73  "dw_z"
  MATLAB Function/1(dq) -> Demux17/1
  Data Store Read24/1 -> MATLAB Function/1(qsc)
  Data Store Read23/1 -> MATLAB Function/2(q_est)
  Data Store Read26/1 -> Sum/1
  Data Store Read25/1 -> Sum/2
  Sum/1 -> Demux18/1
  Demux19/1 -> Bus Creator/74  "TEX_x"
  Demux19/2 -> Bus Creator/75  "TEX_y"
  Demux19/3 -> Bus Creator/76  "TEX_z"
  Data Store Read27/1 -> Demux19/1
  Data Store Read29/1 -> MATLAB Function4/1(CBI)
  Data Store Read28/1 -> MATLAB Function4/2(h_tot_B)
  MATLAB Function4/1(h_tot_I) -> Bus Creator/77

== system ADCS_Simulator/PLANT/ENV ==
  Constant : Constant  Value=ext_torque
  If : If  IfExpression=u1 == 1
  Merge : Merge
  Perturbations Disabled : Subsystem  TreatAsAtomicUnit=on
  Perturbations Enabled : Subsystem  TreatAsAtomicUnit=on
  T_ext : Outport
  wires:
  Constant/1 -> If/1
  If/1 -> Perturbations Enabled/Action
  If/2 -> Perturbations Disabled/Action
  Perturbations Enabled/1(Out1) -> Merge/1
  Perturbations Disabled/1(Out1) -> Merge/2
  Merge/1 -> T_ext/1

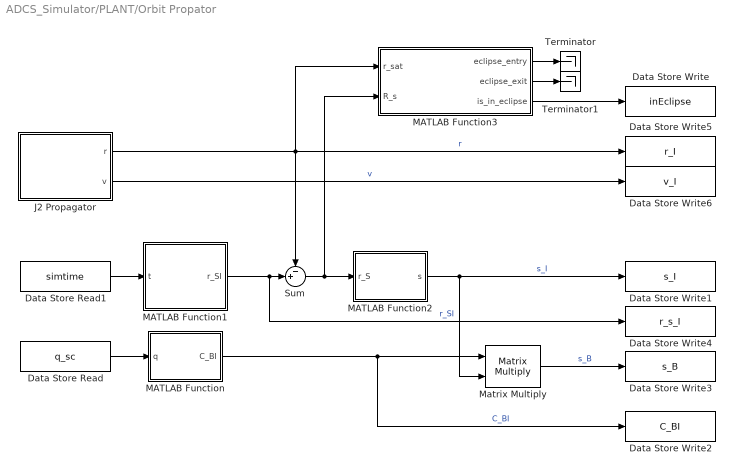
== system ADCS_Simulator/PLANT/Orbit Propator ==
  Data Store Read : DataStoreRead  DataStoreName=q_sc  IndexOptions=Index vector (dialog)  Indices=1  OutputSizes=1
  Data Store Read1 : DataStoreRead  DataStoreName=simtime  IndexOptions=Index vector (dialog)  Indices=1  OutputSizes=1
  Data Store Write : DataStoreWrite  DataStoreName=inEclipse  IndexOptions=Index vector (dialog)  Indices=1  OutputSizes=1
  Data Store Write1 : DataStoreWrite  DataStoreName=s_I  IndexOptions=Index vector (dialog)  Indices=1  OutputSizes=1
  Data Store Write2 : DataStoreWrite  DataStoreName=C_BI  IndexOptions=Index vector (dialog)  Indices=1  OutputSizes=1
  Data Store Write3 : DataStoreWrite  DataStoreName=s_B  IndexOptions=Index vector (dialog)  Indices=1  OutputSizes=1
  Data Store Write4 : DataStoreWrite  DataStoreName=r_s_I  IndexOptions=Index vector (dialog)  Indices=1  OutputSizes=1
  Data Store Write5 : DataStoreWrite  DataStoreName=r_I  IndexOptions=Index vector (dialog)  Indices=1  OutputSizes=1
  Data Store Write6 : DataStoreWrite  DataStoreName=v_I  IndexOptions=Index vector (dialog)  Indices=1  OutputSizes=1
  J2 Propagator : Subsystem
  MATLAB Function : MATLAB Function  TreatAsAtomicUnit=on
  MATLAB Function1 : MATLAB Function  TreatAsAtomicUnit=on
  MATLAB Function2 : MATLAB Function  TreatAsAtomicUnit=on
  MATLAB Function3 : MATLAB Function  TreatAsAtomicUnit=on
  Matrix Multiply : Product  Multiplication=Matrix(*)
  Sum : Sum  Inputs=-+|
  Terminator : Terminator
  Terminator1 : Terminator
  wires:
  MATLAB Function/1(C_BI) -> Data Store Write2/1, Matrix Multiply/1  "C_BI"
  MATLAB Function2/1(s) -> Data Store Write1/1, Matrix Multiply/2  "s_I"
  J2 Propagator/1(r) -> MATLAB Function3/1(r_sat), Sum/1, Data Store Write5/1  "r"
  Data Store Read/1 -> MATLAB Function/1(q)
  Matrix Multiply/1 -> Data Store Write3/1  "s_B"
  J2 Propagator/2(v) -> Data Store Write6/1  "v"
  Data Store Read1/1 -> MATLAB Function1/1(t)
  MATLAB Function1/1(r_SI) -> Data Store Write4/1, Sum/2  "r_SI"
  MATLAB Function3/2(eclipse_exit) -> Terminator1/1
  Sum/1 -> MATLAB Function3/2(R_s), MATLAB Function2/1(r_S)
  MATLAB Function3/1(eclipse_entry) -> Terminator/1
  MATLAB Function3/3(is_in_eclipse) -> Data Store Write/1

== system ADCS_Simulator/PLANT/Spacecraft Dynamics ==
  h_w : Inport
  T_ext : Inport  Port=2
  T_Bdot : Inport  Port=3
  Data Store Write : DataStoreWrite  DataStoreName=h_tot_B  IndexOptions=Index vector (dialog)  Indices=1  OutputSizes=1
  Integrator2 : Integrator  InitialCondition=J_body * [wB_1; wB_2; wB_3]*(pi/180)
  MATLAB Function1 : MATLAB Function  TreatAsAtomicUnit=on
  Reshape : Reshape  OutputDimensionality=Column vector (2-D)  OutputDimensions=[3,1]
  Scope : Scope
      settings: ActiveDisplayYMinimum=-4.3527039546372842E-7  ActiveDisplayYMaximum=4.1195292762308163E-7
  Sum2 : Sum
  w_b : Outport
  wires:
  h_w/1 -> Reshape/1
  T_ext/1 -> Scope/1, Sum2/1
  T_Bdot/1 -> Sum2/2
  Sum2/1 -> MATLAB Function1/2(T_b)
  Reshape/1 -> MATLAB Function1/3(h_w)
  MATLAB Function1/1(h_tot_dot) -> Integrator2/1
  Integrator2/1 -> Data Store Write/1, MATLAB Function1/1(h_tot)
  MATLAB Function1/2(w_b) -> w_b/1

== system ADCS_Simulator/PLANT/Spacecraft Kinematics ==
  note: $\dot \mathbf \epsilon = \frac{1}{2} \left( \eta \ \mathbf I_{3\times3} + \mathbf\epsilon ^{\times} \right) \\ \dot \eta = - \frac{1}{2} \left(\mathbf \epsilon ^{\mathrm{T}} \ \mathbf\omega \right)$
  w : Inport
  Integrator2 : Integrator  InitialCondition=[q1_ini; q2_ini; q3_ini; q4_ini]
  MATLAB Function1 : MATLAB Function  TreatAsAtomicUnit=on
  Quaternion Normalize1 : MATLAB Function  TreatAsAtomicUnit=on
  q : Outport
  wires:
  w/1 -> MATLAB Function1/2(w)
  MATLAB Function1/1(q_dot) -> Integrator2/1
  Integrator2/1 -> Quaternion Normalize1/1(q), MATLAB Function1/1(q)  "q"
  Quaternion Normalize1/1(q_norm) -> q/1

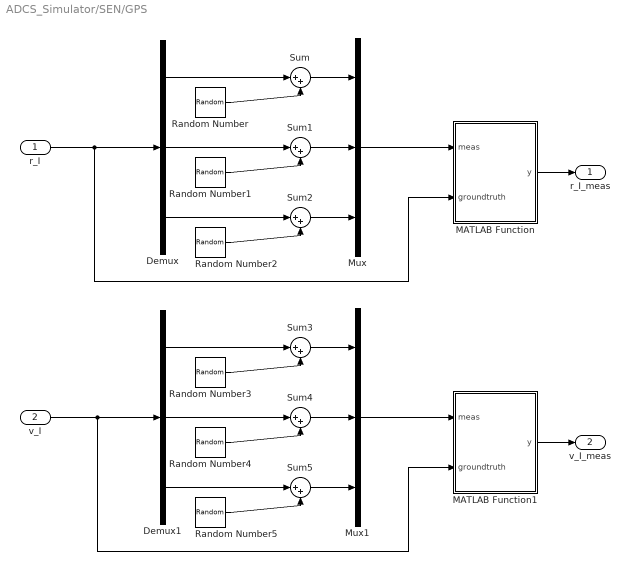
== system ADCS_Simulator/SEN/GPS ==
  r_I : Inport
  v_I : Inport  Port=2
  Demux : Demux  Outputs=3
  Demux1 : Demux  Outputs=3
  MATLAB Function : MATLAB Function  TreatAsAtomicUnit=on
  MATLAB Function1 : MATLAB Function  TreatAsAtomicUnit=on
  Mux : Mux  Inputs=3
  Mux1 : Mux  Inputs=3
  Random Number{,1..5} (6 alike) : RandomNumber  Variance=sigmaGPS^2  Seed=123  SampleTime=1
  Sum{,1..5} (6 alike) : Sum  Inputs=|++
  r_I_meas : Outport
  v_I_meas : Outport  Port=2
  wires:
  Sum1/1 -> Mux/2
  Random Number1/1 -> Sum1/2
  Mux/1 -> MATLAB Function/1(meas)
  Demux/2 -> Sum1/1
  Demux/1 -> Sum/1
  Demux/3 -> Sum2/1
  Sum/1 -> Mux/1
  Sum2/1 -> Mux/3
  Random Number2/1 -> Sum2/2
  r_I/1 -> MATLAB Function/2(groundtruth), Demux/1
  Random Number/1 -> Sum/2
  Mux1/1 -> MATLAB Function1/1(meas)
  v_I/1 -> MATLAB Function1/2(groundtruth), Demux1/1
  Random Number3/1 -> Sum3/2
  Sum4/1 -> Mux1/2
  Sum5/1 -> Mux1/3
  Random Number5/1 -> Sum5/2
  Demux1/1 -> Sum3/1
  Sum3/1 -> Mux1/1
  Random Number4/1 -> Sum4/2
  Demux1/2 -> Sum4/1
  Demux1/3 -> Sum5/1
  MATLAB Function/1(y) -> r_I_meas/1
  MATLAB Function1/1(y) -> v_I_meas/1

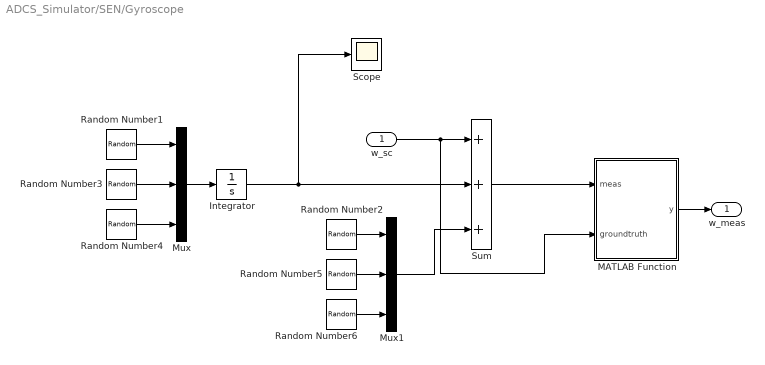
== system ADCS_Simulator/SEN/Gyroscope ==
  w_sc : Inport
  Integrator : Integrator  InitialCondition=1e-09*ones(3,1)
  MATLAB Function : MATLAB Function  TreatAsAtomicUnit=on
  Mux : Mux  Inputs=3
  Mux1 : Mux  Inputs=3
  Random Number1 : RandomNumber  Variance=sigma_b^2  SampleTime=1
  Random Number2 : RandomNumber  Variance=sigma_g^2  SampleTime=1
  Random Number3 : RandomNumber  Variance=sigma_b^2  SampleTime=1
  Random Number4 : RandomNumber  Variance=sigma_b^2  SampleTime=1
  Random Number5 : RandomNumber  Variance=sigma_g^2  SampleTime=1
  Random Number6 : RandomNumber  Variance=sigma_g^2  SampleTime=1
  Scope : Scope
      settings: ActiveDisplayYMinimum=-1  ActiveDisplayYMaximum=1  DataLoggingVariableName=ScopeData2
  Sum : Sum  Inputs=+++
  w_meas : Outport
  wires:
  w_sc/1 -> MATLAB Function/2(groundtruth), Sum/1
  Mux/1 -> Integrator/1
  Random Number1/1 -> Mux/1
  Integrator/1 -> Scope/1, Sum/2
  Mux1/1 -> Sum/3
  Sum/1 -> MATLAB Function/1(meas)
  MATLAB Function/1(y) -> w_meas/1
  Random Number3/1 -> Mux/2
  Random Number4/1 -> Mux/3
  Random Number2/1 -> Mux1/1
  Random Number5/1 -> Mux1/2
  Random Number6/1 -> Mux1/3

== system ADCS_Simulator/SEN/Magnetometer ==
  B_b : Inport
  Demux : Demux  Outputs=3
  MATLAB Function : MATLAB Function  TreatAsAtomicUnit=on
  Mux : Mux  Inputs=3
  Random Number : RandomNumber  Variance=sigma_B^2  Seed=123  SampleTime=1
  Random Number1 : RandomNumber  Variance=sigma_B^2  Seed=123  SampleTime=1
  Random Number2 : RandomNumber  Variance=sigma_B^2  Seed=123  SampleTime=1
  Sum : Sum  Inputs=|++
  Sum1 : Sum  Inputs=|++
  Sum2 : Sum  Inputs=|++
  B_meas : Outport
  wires:
  Mux/1 -> MATLAB Function/1(meas)
  Sum2/1 -> Mux/3
  Random Number/1 -> Sum/2
  Random Number1/1 -> Sum1/2
  Demux/3 -> Sum2/1
  Demux/2 -> Sum1/1
  Sum1/1 -> Mux/2
  Demux/1 -> Sum/1
  Sum/1 -> Mux/1
  Random Number2/1 -> Sum2/2
  MATLAB Function/1(y) -> B_meas/1
  B_b/1 -> MATLAB Function/2(groundtruth), Demux/1

== system ADCS_Simulator/SEN/Sun Sensor ==
  note: This assumes that the sun sensor reference frame coincides
      | with the sc body reference frame
  s_B : Inport
  Data Store Read6 : DataStoreRead  DataStoreName=inEclipse  IndexOptions=Index vector (dialog)  Indices=1  OutputSizes=1
  Demux : Demux  Outputs=3
  MATLAB Function : MATLAB Function  TreatAsAtomicUnit=on
  Mux : Mux  Inputs=3
  Random Number : RandomNumber  Variance=sigma_S^2  SampleTime=1
  Random Number1 : RandomNumber  Variance=sigma_S^2  SampleTime=1
  Random Number2 : RandomNumber  Variance=sigma_S^2  SampleTime=1
  Sum : Sum  Inputs=|++
  Sum1 : Sum  Inputs=|++
  Sum2 : Sum  Inputs=|++
  s_B_meas : Outport
  wires:
  Demux/1 -> Sum/1
  Random Number/1 -> Sum/2
  Demux/2 -> Sum1/1
  Random Number1/1 -> Sum1/2
  Demux/3 -> Sum2/1
  Random Number2/1 -> Sum2/2
  Sum/1 -> Mux/1
  Sum1/1 -> Mux/2
  Sum2/1 -> Mux/3
  s_B/1 -> MATLAB Function/2(groundtruth), Demux/1
  Mux/1 -> MATLAB Function/1(meas)
  Data Store Read6/1 -> MATLAB Function/3(inEclipse)
  MATLAB Function/1(y) -> s_B_meas/1

== system ADCS_Simulator/GNC/Control/Bdot ==
  Action Port : ActionPort  ActionPortLabel=elseif(u1 == 2)
  Bus Creator : BusCreator  Inputs=2
  Controller : MATLAB Function  TreatAsAtomicUnit=on
  Data Store Read9 : DataStoreRead  DataStoreName=b_B_meas  IndexOptions=Index vector (dialog)  Indices=1  OutputSizes=1
  Gain : Gain  Gain=1e-09
  cmd : Outport
  wires:
  Data Store Read9/1 -> Gain/1
  Gain/1 -> Controller/1(B_meas)
  Bus Creator/1 -> cmd/1
  Controller/2(m_cmd) -> Bus Creator/2  "m_cmd"
  Controller/1(T_w) -> Bus Creator/1  "T_cmd"

== system ADCS_Simulator/GNC/Control/Desaturation ==
  Action Port : ActionPort  ActionPortLabel=elseif( u1 == 4)
  Bus Creator : BusCreator  Inputs=2
  Controller : MATLAB Function  TreatAsAtomicUnit=on
  Data Store Read : DataStoreRead  DataStoreName=w_err  IndexOptions=Index vector (dialog)  Indices=1  OutputSizes=1
  Data Store Read1 : DataStoreRead  DataStoreName=w_est  IndexOptions=Index vector (dialog)  Indices=1  OutputSizes=1
  Data Store Read14 : DataStoreRead  DataStoreName=h_wheels  IndexOptions=Index vector (dialog)  Indices=1  OutputSizes=1
  Data Store Read2 : DataStoreRead  DataStoreName=simtime  IndexOptions=Index vector (dialog)  Indices=1  OutputSizes=1
  Data Store Read4 : DataStoreRead  DataStoreName=q_err  IndexOptions=Index vector (dialog)  Indices=1  OutputSizes=1
  Data Store Read9 : DataStoreRead  DataStoreName=b_B_meas  IndexOptions=Index vector (dialog)  Indices=1  OutputSizes=1
  Gain : Gain  Gain=1e-09
  Reshape : Reshape  OutputDimensionality=Column vector (2-D)
  cmd : Outport
  wires:
  Bus Creator/1 -> cmd/1
  Controller/1(T_w) -> Bus Creator/1  "T_cmd"
  Controller/2(M) -> Bus Creator/2  "m_cmd"
  Gain/1 -> Controller/4(B_meas)
  Data Store Read/1 -> Reshape/1
  Data Store Read9/1 -> Gain/1
  Data Store Read1/1 -> Controller/1(w)
  Data Store Read14/1 -> Controller/5(h_w)
  Data Store Read2/1 -> Controller/6(t)
  Reshape/1 -> Controller/3(w_error)
  Data Store Read4/1 -> Controller/2(q_error)

== system ADCS_Simulator/GNC/Control/Detumble ==
  Action Port : ActionPort  ActionPortLabel=elseif( u1 == 3)
  Bus Creator : BusCreator  Inputs=2
  Controller : MATLAB Function  TreatAsAtomicUnit=on
  Data Store Read : DataStoreRead  DataStoreName=w_err  IndexOptions=Index vector (dialog)  Indices=1  OutputSizes=1
  Data Store Read1 : DataStoreRead  DataStoreName=w_est  IndexOptions=Index vector (dialog)  Indices=1  OutputSizes=1
  Data Store Read4 : DataStoreRead  DataStoreName=q_err  IndexOptions=Index vector (dialog)  Indices=1  OutputSizes=1
  Data Store Read9 : DataStoreRead  DataStoreName=b_B_meas  IndexOptions=Index vector (dialog)  Indices=1  OutputSizes=1
  Data Store Write4 : DataStoreWrite  DataStoreName=enableFilter  IndexOptions=Index vector (dialog)  Indices=1  OutputSizes=1
  Gain : Gain  Gain=1e-09
  Scope : Scope
      settings: ActiveDisplayYMinimum=-0.125  ActiveDisplayYMaximum=1.125
  cmd : Outport
  wires:
  Bus Creator/1 -> cmd/1
  Controller/2(M) -> Bus Creator/2  "m_cmd"
  Controller/1(T_w) -> Bus Creator/1  "T_cmd"
  Data Store Read9/1 -> Gain/1
  Gain/1 -> Controller/4(B_meas)
  Data Store Read1/1 -> Controller/1(w)
  Data Store Read/1 -> Controller/3(w_error)
  Data Store Read4/1 -> Controller/2(q_error)
  Controller/3(enableFilter) -> Scope/1, Data Store Write4/1

== system ADCS_Simulator/GNC/Control/No Control ==
  Action Port : ActionPort  ActionPortLabel=else
  Bus Creator : BusCreator  Inputs=2
  MATLAB Function : MATLAB Function  TreatAsAtomicUnit=on
  cmd : Outport
  wires:
  MATLAB Function/1(Tcmd) -> Bus Creator/1  "T_cmd"
  MATLAB Function/2(m_cmd) -> Bus Creator/2  "m_cmd"
  Bus Creator/1 -> cmd/1

== system ADCS_Simulator/GNC/Control/PD  ==
  note: PD Control
  Action Port : ActionPort  ActionPortLabel=if(u1 == 1)
  Bus Creator : BusCreator  Inputs=2
  Data Store Read : DataStoreRead  DataStoreName=w_err  IndexOptions=Index vector (dialog)  Indices=1  OutputSizes=1
  Data Store Read1 : DataStoreRead  DataStoreName=w_est  IndexOptions=Index vector (dialog)  Indices=1  OutputSizes=1
  Data Store Read4 : DataStoreRead  DataStoreName=q_err  IndexOptions=Index vector (dialog)  Indices=1  OutputSizes=1
  PD Controller : MATLAB Function  TreatAsAtomicUnit=on
  cmd : Outport
  wires:
  Data Store Read1/1 -> PD Controller/1(w)
  Data Store Read4/1 -> PD Controller/2(q_error)
  Data Store Read/1 -> PD Controller/3(w_error)
  Bus Creator/1 -> cmd/1
  PD Controller/1(T_w) -> Bus Creator/1  "T_cmd"
  PD Controller/2(M) -> Bus Creator/2  "m_cmd"

== system ADCS_Simulator/GNC/Guidance/Error ==
  q_des : Inport
  w_des : Inport  Port=2
  w_body : Inport  Port=3
  q_body : Inport  Port=4
  Error Quaternion : MATLAB Function  TreatAsAtomicUnit=on
  MATLAB Function : MATLAB Function  TreatAsAtomicUnit=on
  Scope{,1..3} (4 alike) : Scope
      Scope settings: Title=Pointing Error  ShowGrid=off  ActiveDisplayYMinimum=-30.396747339748117  ActiveDisplayYMaximum=42.247837440777545  YLabel=\theta_{e} (deg)
      Scope1 settings: Title=Pointing Error  ShowGrid=off  ActiveDisplayYMinimum=-0.0048961039434763255  ActiveDisplayYMaximum=0.0065575778487023933  YLabel=\theta_{e} (deg)
      Scope2 settings: ActiveDisplayYMinimum=-0.1286  ActiveDisplayYMaximum=1.1254
      Scope3 settings: ActiveDisplayYMinimum=-1.13656  ActiveDisplayYMaximum=1.16025  DataLoggingVariableName=ScopeData2
  Sum : Sum  Inputs=|-+
  w_error : Outport
  q_error : Outport  Port=2
  wires:
  q_des/1 -> Error Quaternion/2(q_d)
  q_body/1 -> Scope3/1, Error Quaternion/1(q)
  w_body/1 -> Sum/1
  w_des/1 -> Sum/2
  Sum/1 -> Scope1/1, w_error/1
  MATLAB Function/1(theta_e) -> Scope/1
  Error Quaternion/1(delta_q) -> MATLAB Function/1(q_error), Scope2/1, q_error/1
